simulink model "raspiAutopilotControlSystem"  (R2017b)
settings: Solver=ode5  StartTime=0.0  StopTime=inf  RelTol=1e-3  EnableMultiTasking=on
undefined symbols (not defined in the file): ap, env, sensors
libraries: etargetslib x2, simulink_extras x2, embdlinuxlib x2, mbdriLib x1
settings Model: ParamWorkspaceSource=ReferencedWorkspace  Creator=mlizarra  LastModifiedBy=mboyle
settings SolverCC: PositivePriorityOrder=on  AutoInsertRateTranBlk=on
settings DataIOCC: SaveOutput=off  DSMLogging=off  SaveTime=off  ReturnWorkspaceOutputs=on
settings OptimizationCC: DefaultParameterBehavior=Inlined  UseDivisionForNetSlopeComputation=UseDivisionForReciprocalsOfIntegersOnly  DefaultUnderspecifiedDataType=single  InlineInvariantSignals=on  PassReuseOutputArgsAs=Individual arguments  StateBitsets=on  DataBitsets=on  ZeroExternalMemoryAtStartup=off  ZeroInternalMemoryAtStartup=off  EfficientFloat2IntCast=on  LifeSpan=1  MaxStackSize=64
settings DebuggingCC: SignalInfNanChecking=warning  AlgebraicLoopMsg=error  ParameterPrecisionLossMsg=none  UniqueDataStoreMsg=error  AssertControl=DisableAll  SFUnexpectedBacktrackingDiag=warning  SFNoUnconditionalDefaultTransitionDiag=warning  SFExecutionAtInitializationDiag=none
settings HardwareCC: ProdBitPerPointer=32  ProdBitPerSizeT=32  ProdBitPerPtrDiffT=32  ProdLargestAtomicInteger=Long  ProdLargestAtomicFloat=Double  ProdWordSize=32  ProdHWDeviceType=ARM Compatible->ARM Cortex
settings SFSimCC: SimGenImportedTypeDefs=on  MATLABDynamicMemAlloc=off
settings RTWCC: SystemTargetFile=ert.tlc  HardwareBoard=Raspberry Pi  TemplateMakefile=ert_default_tmf  PostCodeGenCommand=add_header_files(h);  GenerateReport=on  CustomInclude=../src  Toolchain=GNU GCC Raspberry Pi  IncludeHyperlinkInReport=on  LaunchReport=on  PortableWordSizes=on  GenerateTraceInfo=on  GenerateTraceReport=on  GenerateTraceReportSl=on  GenerateTraceReportSf=on  GenerateTraceReportEml=on
settings CodeAppCC: ForceParamTrailComments=on  IgnoreCustomStorageClasses=off  IgnoreTestpoints=on  OperatorAnnotations=on  SimulinkDataObjDesc=on  SFDataObjDesc=on  MATLABFcnDesc=on  InsertBlockDesc=on  MATLABSourceComments=on
settings ERTTargetCC: TargetLangStandard=C99 (ISO)  CodeReplacementLibrary=GNU C99 extensions  SupportNonFinite=off  SupportVariableSizeSignals=on  InlinedParameterPlacement=NonHierarchical
settings ConfigComp: CovSaveCumulativeToWorkspaceVar=on

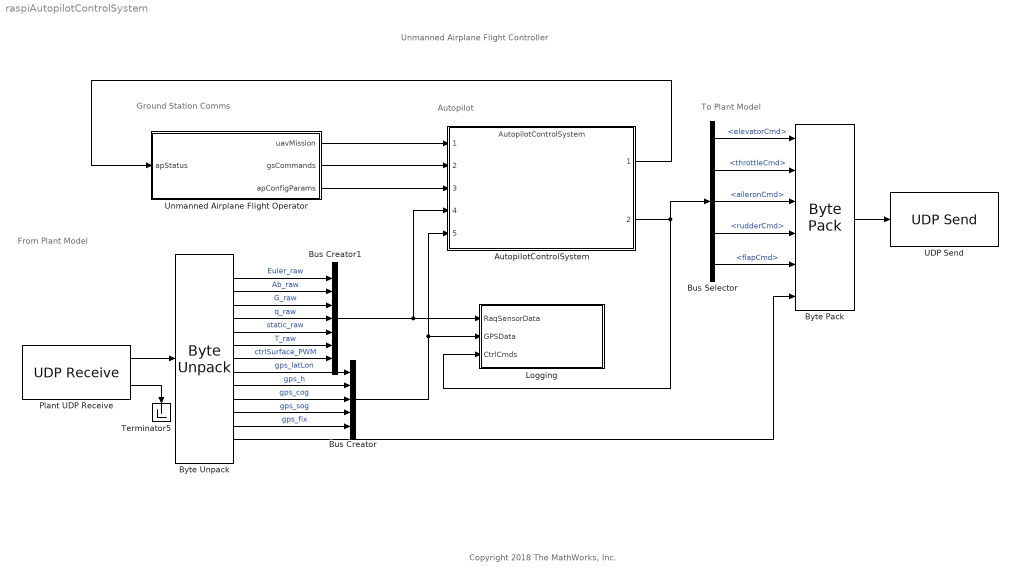
== system raspiAutopilotControlSystem ==
  note: To Plant Model
  note: From Plant Model
  note: Unmanned Airplane Flight Controller
  note: Ground Station Comms
  note: Autopilot
  note: Copyright 2018 The MathWorks, Inc.
  AutopilotControlSystem : ModelReference  ModelNameDialog=AutopilotControlSystem  SimulationMode=Normal  ModelReferenceVersion=1.356
  Bus Creator : BusCreator  Inputs=5  OutDataTypeStr=Bus: gpsReading
  Bus Creator1 : BusCreator  Inputs=7  OutDataTypeStr=Bus: rawSensorDataBus
  Bus Selector : BusSelector  OutputSignals=elevatorCmd,throttleCmd,aileronCmd,rudderCmd,flapCmd
  Byte Pack : etargetslib/Byte Pack  datatypes={'single', 'single','single', 'single','single','double'}  byteAlign=1
  Byte Unpack : etargetslib/Byte Unpack  dimensions={[3],[3],[3],1,1,1,[5],[2],1,1,1,1,1}  datatypes={'int16','int16','int16','uint16','uint16','int16','int16','single','single','single','single','uint8','double'}  byteAlign=1
  Logging : Subsystem
  Plant UDP Receive : embdlinuxlib/UDP Receive  localURL='0.0.0.0'  localPort=25001  remoteURL='0.0.0.0'  remotePort=-1  recvBufferSize=8192  signalDatatype=uint8  dims=63  isVarSize=off  showBlockingTime=off  blockingTime=0  sampletime=0.01  blockPlatform=Raspberry Pi
      settings: SourceProductName=Simulink Support Package for Raspberry Pi Hardware  SourceProductBaseCode=RASPPI
  Terminator5 : Terminator
  UDP Send : embdlinuxlib/UDP Send  remoteURL='10.10.10.6'  remotePort=25000  localURL='255.255.255.255'  localPortSource=Automatically determine  localPort=-1  sampletime=-1  blockPlatform=Raspberry Pi  separateLengthPort=0
      settings: SourceProductName=Simulink Support Package for Raspberry Pi Hardware  SourceProductBaseCode=RASPPI
  "Unmanned Airplane Flight Operator " : Subsystem
  wires:
  "Unmanned Airplane Flight Operator "/2(gsCommands) -> AutopilotControlSystem/2
  "Unmanned Airplane Flight Operator "/3(apConfigParams) -> AutopilotControlSystem/3
  AutopilotControlSystem/1 -> "Unmanned Airplane Flight Operator "/1(apStatus)
  "Unmanned Airplane Flight Operator "/1(uavMission) -> AutopilotControlSystem/1
  Plant UDP Receive/1 -> Byte Unpack/1
  Plant UDP Receive/2 -> Terminator5/1
  Byte Pack/1 -> UDP Send/1
  Bus Selector/1 -> Byte Pack/1  "<elevatorCmd>"
  Bus Selector/2 -> Byte Pack/2  "<throttleCmd>"
  Bus Selector/3 -> Byte Pack/3  "<aileronCmd>"
  Bus Selector/4 -> Byte Pack/4  "<rudderCmd>"
  Bus Selector/5 -> Byte Pack/5  "<flapCmd>"
  Byte Unpack/1 -> Bus Creator1/1  "Euler_raw"
  Byte Unpack/4 -> Bus Creator1/4  "q_raw"
  Byte Unpack/7 -> Bus Creator1/7  "ctrlSurface_PWM"
  Byte Unpack/6 -> Bus Creator1/6  "T_raw"
  Byte Unpack/3 -> Bus Creator1/3  "G_raw"
  Byte Unpack/5 -> Bus Creator1/5  "static_raw"
  Byte Unpack/2 -> Bus Creator1/2  "Ab_raw"
  Byte Unpack/12 -> Bus Creator/5  "gps_fix"
  Byte Unpack/11 -> Bus Creator/4  "gps_sog"
  Byte Unpack/10 -> Bus Creator/3  "gps_cog"
  Byte Unpack/9 -> Bus Creator/2  "gps_h"
  Byte Unpack/8 -> Bus Creator/1  "gps_latLon"
  Bus Creator1/1 -> AutopilotControlSystem/4, Logging/1(RaqSensorData)
  Bus Creator/1 -> AutopilotControlSystem/5, Logging/2(GPSData)
  AutopilotControlSystem/2 -> Logging/3(CtrlCmds), Bus Selector/1
  Byte Unpack/13 -> Byte Pack/6

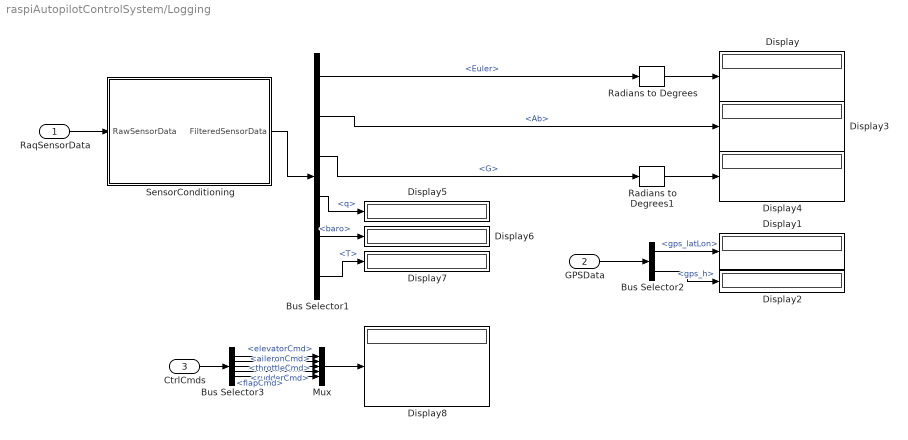
== system raspiAutopilotControlSystem/Logging ==
  RaqSensorData : Inport
  GPSData : Inport  Port=2
  CtrlCmds : Inport  Port=3
  Bus Selector1 : BusSelector  OutputSignals=Euler,Ab,G,q,baro,T
  Bus Selector2 : BusSelector  OutputSignals=gps_latLon,gps_h
  Bus Selector3 : BusSelector  OutputSignals=elevatorCmd,throttleCmd,aileronCmd,rudderCmd,flapCmd
  Display{,1..8} (9 alike) : Display
  Mux : Mux  Inputs=5
  Radians to Degrees : simulink_extras/Transformations/Radians to Degrees
  Radians to Degrees1 : simulink_extras/Transformations/Radians to Degrees
  SensorConditioning : Subsystem  TreatAsAtomicUnit=on
  wires:
  Bus Selector2/1 -> Display1/1  "<gps_latLon>"
  Bus Selector1/1 -> Radians to Degrees/1  "<Euler>"
  GPSData/1 -> Bus Selector2/1
  Bus Selector2/2 -> Display2/1  "<gps_h>"
  RaqSensorData/1 -> SensorConditioning/1(RawSensorData)
  SensorConditioning/1(FilteredSensorData) -> Bus Selector1/1
  Bus Selector1/2 -> Display3/1  "<Ab>"
  Bus Selector1/3 -> Radians to Degrees1/1  "<G>"
  Bus Selector1/4 -> Display5/1  "<q>"
  Bus Selector1/5 -> Display6/1  "<baro>"
  Bus Selector1/6 -> Display7/1  "<T>"
  Radians to Degrees/1 -> Display/1
  Radians to Degrees1/1 -> Display4/1
  CtrlCmds/1 -> Bus Selector3/1
  Bus Selector3/1 -> Mux/1  "<elevatorCmd>"
  Bus Selector3/2 -> Mux/2  "<throttleCmd>"
  Bus Selector3/3 -> Mux/3  "<aileronCmd>"
  Bus Selector3/4 -> Mux/4  "<rudderCmd>"
  Bus Selector3/5 -> Mux/5  "<flapCmd>"
  Mux/1 -> Display8/1

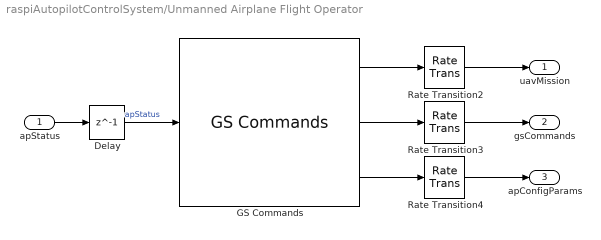
== system raspiAutopilotControlSystem/Unmanned Airplane Flight Operator  ==
  apStatus : Inport  OutDataTypeStr=Bus: apStatusBus
  Delay : Delay  DelayLength=1
  "GS Commands " : mbdriLib/Utilities/GS Commands 
  Rate Transition2 : RateTransition  OutPortSampleTime=ap.apSampleTime
  Rate Transition3 : RateTransition  OutPortSampleTime=ap.apSampleTime
  Rate Transition4 : RateTransition  OutPortSampleTime=ap.apSampleTime
  uavMission : Outport  OutDataTypeStr=Bus: waypoint
  gsCommands : Outport  Port=2  OutDataTypeStr=Bus: gsCommandsBus
  apConfigParams : Outport  Port=3  OutDataTypeStr=Bus: apConfigParamsBus
  wires:
  Rate Transition2/1 -> uavMission/1
  "GS Commands "/3 -> Rate Transition4/1
  apStatus/1 -> Delay/1
  "GS Commands "/2 -> Rate Transition3/1
  Delay/1 -> "GS Commands "/1  "apStatus"
  "GS Commands "/1 -> Rate Transition2/1
  Rate Transition4/1 -> apConfigParams/1
  Rate Transition3/1 -> gsCommands/1

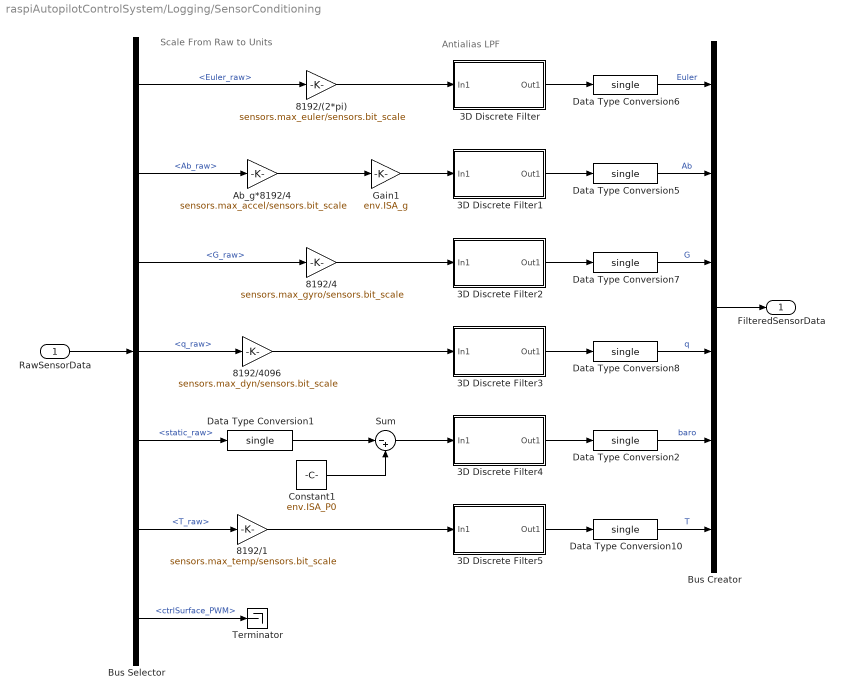
== system raspiAutopilotControlSystem/Logging/SensorConditioning ==
  note: Antialias LPF
  note: Scale From Raw to Units
  RawSensorData : Inport
  3D Discrete Filter : Subsystem  RTWFcnName=TustinFilter3D  mask{bw=sensors.antialiasBW, TSample=ap.apSampleTime}
      mask prompts: bw "Bandwith (Hz)"; TSample "Sample Time"
      mask init:
      | tau = 1/(2*pi*bw);
      | zval = [];
      | pval = -1/tau;
      | kval = 1/tau;
      | 
      | set_param(gcb,'AttributesFormatString', ['Fc = ' num2str(bw)]);
      settings: AttributesFormatString=Fc = 40  RTWFcnNameOpts=User specified  RTWFileNameOpts=Use function name
      mask Display:
      | droots(zval,pval,kval)
      | port_label('input',1,'3D')
  3D Discrete Filter1 : Subsystem  RTWFcnName=TustinFilter3D  mask{bw=sensors.antialiasBW, TSample=ap.apSampleTime}
      mask prompts: bw "Bandwith (Hz)"; TSample "Sample Time"
      mask init:
      | tau = 1/(2*pi*bw);
      | zval = [];
      | pval = -1/tau;
      | kval = 1/tau;
      | 
      | set_param(gcb,'AttributesFormatString', ['Fc = ' num2str(bw)]);
      settings: AttributesFormatString=Fc = 40  RTWFcnNameOpts=User specified  RTWFileNameOpts=Use function name
      mask Display:
      | droots(zval,pval,kval)
      | port_label('input',1,'3D')
  3D Discrete Filter2 : Subsystem  RTWFcnName=TustinFilter3D  mask{bw=sensors.antialiasBW, TSample=ap.apSampleTime}
      mask prompts: bw "Bandwith (Hz)"; TSample "Sample Time"
      mask init:
      | tau = 1/(2*pi*bw);
      | zval = [];
      | pval = -1/tau;
      | kval = 1/tau;
      | 
      | set_param(gcb,'AttributesFormatString', ['Fc = ' num2str(bw)]);
      settings: AttributesFormatString=Fc = 40  RTWFcnNameOpts=User specified  RTWFileNameOpts=Use function name
      mask Display:
      | droots(zval,pval,kval)
      | port_label('input',1,'3D')
  3D Discrete Filter3 : Subsystem  RTWFcnName=TustinFilter3D  mask{bw=sensors.antialiasBW, TSample=ap.apSampleTime}
      mask prompts: bw "Bandwith (Hz)"; TSample "Sample Time"
      mask init:
      | tau = 1/(2*pi*bw);
      | zval = [];
      | pval = -1/tau;
      | kval = 1/tau;
      | 
      | set_param(gcb,'AttributesFormatString', ['Fc = ' num2str(bw)]);
      settings: AttributesFormatString=Fc = 40  RTWFcnNameOpts=User specified  RTWFileNameOpts=Use function name
      mask Display:
      | droots(zval,pval,kval)
      | port_label('input',1,'1D')
  3D Discrete Filter4 : Subsystem  RTWFcnName=TustinFilter3D  mask{bw=sensors.antialiasBW, TSample=ap.apSampleTime}
      mask prompts: bw "Bandwith (Hz)"; TSample "Sample Time"
      mask init:
      | tau = 1/(2*pi*bw);
      | zval = [];
      | pval = -1/tau;
      | kval = 1/tau;
      | 
      | set_param(gcb,'AttributesFormatString', ['Fc = ' num2str(bw)]);
      settings: AttributesFormatString=Fc = 40  RTWFcnNameOpts=User specified  RTWFileNameOpts=Use function name
      mask Display:
      | droots(zval,pval,kval)
      | port_label('input',1,'1D')
  3D Discrete Filter5 : Subsystem  RTWFcnName=TustinFilter3D  mask{bw=sensors.antialiasBW, TSample=ap.apSampleTime}
      mask prompts: bw "Bandwith (Hz)"; TSample "Sample Time"
      mask init:
      | tau = 1/(2*pi*bw);
      | zval = [];
      | pval = -1/tau;
      | kval = 1/tau;
      | 
      | set_param(gcb,'AttributesFormatString', ['Fc = ' num2str(bw)]);
      settings: AttributesFormatString=Fc = 40  RTWFcnNameOpts=User specified  RTWFileNameOpts=Use function name
      mask Display:
      | droots(zval,pval,kval)
      | port_label('input',1,'1D')
  8192/(2*pi) : Gain  Gain=sensors.max_euler/sensors.bit_scale  OutDataTypeStr=single
      settings: AttributesFormatString=%<Gain>
  8192/1 : Gain  Gain=sensors.max_temp/sensors.bit_scale  OutDataTypeStr=single
      settings: AttributesFormatString=%<Gain>
  8192/4 : Gain  Gain=sensors.max_gyro/sensors.bit_scale  OutDataTypeStr=single
      settings: AttributesFormatString=%<Gain>
  8192/4096 : Gain  Gain=sensors.max_dyn/sensors.bit_scale  OutDataTypeStr=single
      settings: AttributesFormatString=%<Gain>
  Ab_g*8192/4 : Gain  Gain=sensors.max_accel/sensors.bit_scale  OutDataTypeStr=single
      settings: AttributesFormatString=%<Gain>
  Bus Creator : BusCreator  Inputs=6
  Bus Selector : BusSelector  OutputSignals=Euler_raw,Ab_raw,G_raw,q_raw,static_raw,T_raw,ctrlSurface_PWM
  Constant1 : Constant  Value=env.ISA_P0
      settings: AttributesFormatString=%<Value>
  Data Type Conversion{1..2,5..8,10} (7 alike) : DataTypeConversion  OutDataTypeStr=single
  Gain1 : Gain  Gain=env.ISA_g  OutDataTypeStr=single
      settings: AttributesFormatString=%<Gain>
  Sum : Sum  Inputs=|-+
  Terminator : Terminator
  FilteredSensorData : Outport
  wires:
  3D Discrete Filter5/1(Out1) -> Data Type Conversion10/1
  Data Type Conversion2/1 -> Bus Creator/5  "baro"
  3D Discrete Filter4/1(Out1) -> Data Type Conversion2/1
  3D Discrete Filter3/1(Out1) -> Data Type Conversion8/1
  3D Discrete Filter2/1(Out1) -> Data Type Conversion7/1
  3D Discrete Filter1/1(Out1) -> Data Type Conversion5/1
  3D Discrete Filter/1(Out1) -> Data Type Conversion6/1
  Data Type Conversion1/1 -> Sum/1
  Bus Creator/1 -> FilteredSensorData/1
  Gain1/1 -> 3D Discrete Filter1/1(In1)
  Bus Selector/2 -> Ab_g*8192/4/1  "<Ab_raw>"
  RawSensorData/1 -> Bus Selector/1
  Data Type Conversion6/1 -> Bus Creator/1  "Euler"
  Data Type Conversion5/1 -> Bus Creator/2  "Ab"
  Data Type Conversion7/1 -> Bus Creator/3  "G"
  Data Type Conversion8/1 -> Bus Creator/4  "q"
  Sum/1 -> 3D Discrete Filter4/1(In1)
  Data Type Conversion10/1 -> Bus Creator/6  "T"
  Constant1/1 -> Sum/2
  8192/1/1 -> 3D Discrete Filter5/1(In1)
  8192/4096/1 -> 3D Discrete Filter3/1(In1)
  Bus Selector/6 -> 8192/1/1  "<T_raw>"
  Bus Selector/5 -> Data Type Conversion1/1  "<static_raw>"
  Bus Selector/4 -> 8192/4096/1  "<q_raw>"
  Bus Selector/3 -> 8192/4/1  "<G_raw>"
  8192/4/1 -> 3D Discrete Filter2/1(In1)
  8192/(2*pi)/1 -> 3D Discrete Filter/1(In1)
  Ab_g*8192/4/1 -> Gain1/1
  Bus Selector/1 -> 8192/(2*pi)/1  "<Euler_raw>"
  Bus Selector/7 -> Terminator/1  "<ctrlSurface_PWM>"

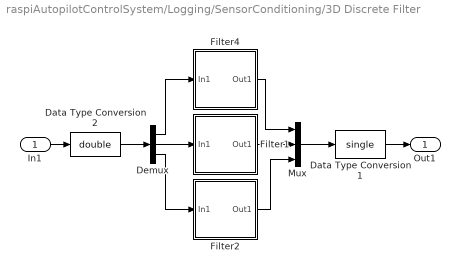
== system raspiAutopilotControlSystem/Logging/SensorConditioning/3D Discrete Filter ==
  In1 : Inport
  Data Type Conversion1 : DataTypeConversion  OutDataTypeStr=single
  Data Type Conversion2 : DataTypeConversion  OutDataTypeStr=double
  Demux : Demux  Outputs=3
  Filter1 : Subsystem  mask{Zeros=zval, Poles=pval, Gain=kval, AbsTol=auto, SampleTime=TSample, method=tustin, Wc=1}
      mask prompts: Zeros "Zeros (enter in s-main:)"; Poles "Poles (enter in s-domain:)"; Gain "Gain (enter in s-domain:)"; AbsTol "Absolute tolerance:"; SampleTime "Sample time:"; Wc "Critical Frequency (Hz):"
      mask init:
      | H = zpk(Zeros, Poles, Gain);
      | Hd = c2d(H, SampleTime, 'tustin');
      | [z, p, g] = zpkdata(Hd);
      | z_d = z{:};
      | p_d = p{:};
      | g_d = g;
      mask TypeOptions method: zoh | foh | tustin | prewarp | matched
      mask Display: droots(Zeros,Poles,Gain)
  Filter2 : Subsystem  mask{Zeros=zval, Poles=pval, Gain=kval, AbsTol=auto, SampleTime=TSample, method=tustin, Wc=1}
      mask prompts: Zeros "Zeros (enter in s-main:)"; Poles "Poles (enter in s-domain:)"; Gain "Gain (enter in s-domain:)"; AbsTol "Absolute tolerance:"; SampleTime "Sample time:"; Wc "Critical Frequency (Hz):"
      mask init:
      | H = zpk(Zeros, Poles, Gain);
      | Hd = c2d(H, SampleTime, 'tustin');
      | [z, p, g] = zpkdata(Hd);
      | z_d = z{:};
      | p_d = p{:};
      | g_d = g;
      mask TypeOptions method: zoh | foh | tustin | prewarp | matched
      mask Display: droots(Zeros,Poles,Gain)
  Filter4 : Subsystem  mask{Zeros=zval, Poles=pval, Gain=kval, AbsTol=auto, SampleTime=TSample, method=tustin, Wc=1}
      mask prompts: Zeros "Zeros (enter in s-main:)"; Poles "Poles (enter in s-domain:)"; Gain "Gain (enter in s-domain:)"; AbsTol "Absolute tolerance:"; SampleTime "Sample time:"; Wc "Critical Frequency (Hz):"
      mask init:
      | H = zpk(Zeros, Poles, Gain);
      | Hd = c2d(H, SampleTime, 'tustin');
      | [z, p, g] = zpkdata(Hd);
      | z_d = z{:};
      | p_d = p{:};
      | g_d = g;
      mask TypeOptions method: zoh | foh | tustin | prewarp | matched
      mask Display: droots(Zeros,Poles,Gain)
  Mux : Mux  Inputs=3
  Out1 : Outport
  wires:
  Data Type Conversion1/1 -> Out1/1
  Data Type Conversion2/1 -> Demux/1
  Demux/1 -> Filter4/1(In1)
  Demux/2 -> Filter1/1(In1)
  Demux/3 -> Filter2/1(In1)
  Filter4/1(Out1) -> Mux/1
  Filter1/1(Out1) -> Mux/2
  Filter2/1(Out1) -> Mux/3
  In1/1 -> Data Type Conversion2/1
  Mux/1 -> Data Type Conversion1/1

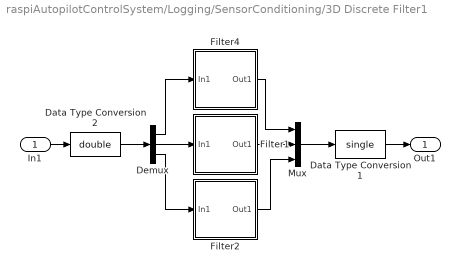
== system raspiAutopilotControlSystem/Logging/SensorConditioning/3D Discrete Filter1 ==
  In1 : Inport
  Data Type Conversion1 : DataTypeConversion  OutDataTypeStr=single
  Data Type Conversion2 : DataTypeConversion  OutDataTypeStr=double
  Demux : Demux  Outputs=3
  Filter1 : Subsystem  mask{Zeros=zval, Poles=pval, Gain=kval, AbsTol=auto, SampleTime=TSample, method=tustin, Wc=1}
      mask prompts: Zeros "Zeros (enter in s-main:)"; Poles "Poles (enter in s-domain:)"; Gain "Gain (enter in s-domain:)"; AbsTol "Absolute tolerance:"; SampleTime "Sample time:"; Wc "Critical Frequency (Hz):"
      mask init:
      | H = zpk(Zeros, Poles, Gain);
      | Hd = c2d(H, SampleTime, 'tustin');
      | [z, p, g] = zpkdata(Hd);
      | z_d = z{:};
      | p_d = p{:};
      | g_d = g;
      mask TypeOptions method: zoh | foh | tustin | prewarp | matched
      mask Display: droots(Zeros,Poles,Gain)
  Filter2 : Subsystem  mask{Zeros=zval, Poles=pval, Gain=kval, AbsTol=auto, SampleTime=TSample, method=tustin, Wc=1}
      mask prompts: Zeros "Zeros (enter in s-main:)"; Poles "Poles (enter in s-domain:)"; Gain "Gain (enter in s-domain:)"; AbsTol "Absolute tolerance:"; SampleTime "Sample time:"; Wc "Critical Frequency (Hz):"
      mask init:
      | H = zpk(Zeros, Poles, Gain);
      | Hd = c2d(H, SampleTime, 'tustin');
      | [z, p, g] = zpkdata(Hd);
      | z_d = z{:};
      | p_d = p{:};
      | g_d = g;
      mask TypeOptions method: zoh | foh | tustin | prewarp | matched
      mask Display: droots(Zeros,Poles,Gain)
  Filter4 : Subsystem  mask{Zeros=zval, Poles=pval, Gain=kval, AbsTol=auto, SampleTime=TSample, method=tustin, Wc=1}
      mask prompts: Zeros "Zeros (enter in s-main:)"; Poles "Poles (enter in s-domain:)"; Gain "Gain (enter in s-domain:)"; AbsTol "Absolute tolerance:"; SampleTime "Sample time:"; Wc "Critical Frequency (Hz):"
      mask init:
      | H = zpk(Zeros, Poles, Gain);
      | Hd = c2d(H, SampleTime, 'tustin');
      | [z, p, g] = zpkdata(Hd);
      | z_d = z{:};
      | p_d = p{:};
      | g_d = g;
      mask TypeOptions method: zoh | foh | tustin | prewarp | matched
      mask Display: droots(Zeros,Poles,Gain)
  Mux : Mux  Inputs=3
  Out1 : Outport
  wires:
  Mux/1 -> Data Type Conversion1/1
  In1/1 -> Data Type Conversion2/1
  Filter2/1(Out1) -> Mux/3
  Filter1/1(Out1) -> Mux/2
  Filter4/1(Out1) -> Mux/1
  Demux/3 -> Filter2/1(In1)
  Demux/2 -> Filter1/1(In1)
  Demux/1 -> Filter4/1(In1)
  Data Type Conversion2/1 -> Demux/1
  Data Type Conversion1/1 -> Out1/1

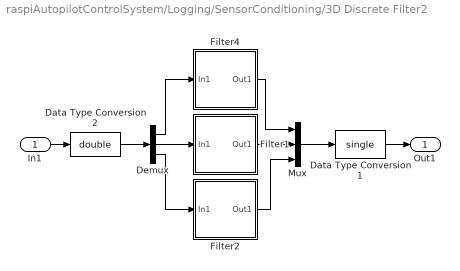
== system raspiAutopilotControlSystem/Logging/SensorConditioning/3D Discrete Filter2 ==
  In1 : Inport
  Data Type Conversion1 : DataTypeConversion  OutDataTypeStr=single
  Data Type Conversion2 : DataTypeConversion  OutDataTypeStr=double
  Demux : Demux  Outputs=3
  Filter1 : Subsystem  mask{Zeros=zval, Poles=pval, Gain=kval, AbsTol=auto, SampleTime=TSample, method=tustin, Wc=1}
      mask prompts: Zeros "Zeros (enter in s-main:)"; Poles "Poles (enter in s-domain:)"; Gain "Gain (enter in s-domain:)"; AbsTol "Absolute tolerance:"; SampleTime "Sample time:"; Wc "Critical Frequency (Hz):"
      mask init:
      | H = zpk(Zeros, Poles, Gain);
      | Hd = c2d(H, SampleTime, 'tustin');
      | [z, p, g] = zpkdata(Hd);
      | z_d = z{:};
      | p_d = p{:};
      | g_d = g;
      mask TypeOptions method: zoh | foh | tustin | prewarp | matched
      mask Display: droots(Zeros,Poles,Gain)
  Filter2 : Subsystem  mask{Zeros=zval, Poles=pval, Gain=kval, AbsTol=auto, SampleTime=TSample, method=tustin, Wc=1}
      mask prompts: Zeros "Zeros (enter in s-main:)"; Poles "Poles (enter in s-domain:)"; Gain "Gain (enter in s-domain:)"; AbsTol "Absolute tolerance:"; SampleTime "Sample time:"; Wc "Critical Frequency (Hz):"
      mask init:
      | H = zpk(Zeros, Poles, Gain);
      | Hd = c2d(H, SampleTime, 'tustin');
      | [z, p, g] = zpkdata(Hd);
      | z_d = z{:};
      | p_d = p{:};
      | g_d = g;
      mask TypeOptions method: zoh | foh | tustin | prewarp | matched
      mask Display: droots(Zeros,Poles,Gain)
  Filter4 : Subsystem  mask{Zeros=zval, Poles=pval, Gain=kval, AbsTol=auto, SampleTime=TSample, method=tustin, Wc=1}
      mask prompts: Zeros "Zeros (enter in s-main:)"; Poles "Poles (enter in s-domain:)"; Gain "Gain (enter in s-domain:)"; AbsTol "Absolute tolerance:"; SampleTime "Sample time:"; Wc "Critical Frequency (Hz):"
      mask init:
      | H = zpk(Zeros, Poles, Gain);
      | Hd = c2d(H, SampleTime, 'tustin');
      | [z, p, g] = zpkdata(Hd);
      | z_d = z{:};
      | p_d = p{:};
      | g_d = g;
      mask TypeOptions method: zoh | foh | tustin | prewarp | matched
      mask Display: droots(Zeros,Poles,Gain)
  Mux : Mux  Inputs=3
  Out1 : Outport
  wires:
  Data Type Conversion1/1 -> Out1/1
  Data Type Conversion2/1 -> Demux/1
  Demux/1 -> Filter4/1(In1)
  Demux/2 -> Filter1/1(In1)
  Demux/3 -> Filter2/1(In1)
  Filter4/1(Out1) -> Mux/1
  Filter1/1(Out1) -> Mux/2
  Filter2/1(Out1) -> Mux/3
  In1/1 -> Data Type Conversion2/1
  Mux/1 -> Data Type Conversion1/1

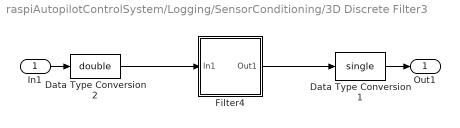
== system raspiAutopilotControlSystem/Logging/SensorConditioning/3D Discrete Filter3 ==
  In1 : Inport
  Data Type Conversion1 : DataTypeConversion  OutDataTypeStr=single
  Data Type Conversion2 : DataTypeConversion  OutDataTypeStr=double
  Filter4 : Subsystem  mask{Zeros=zval, Poles=pval, Gain=kval, AbsTol=auto, SampleTime=TSample, method=tustin, Wc=1}
      mask prompts: Zeros "Zeros (enter in s-main:)"; Poles "Poles (enter in s-domain:)"; Gain "Gain (enter in s-domain:)"; AbsTol "Absolute tolerance:"; SampleTime "Sample time:"; Wc "Critical Frequency (Hz):"
      mask init:
      | H = zpk(Zeros, Poles, Gain);
      | Hd = c2d(H, SampleTime, 'tustin');
      | [z, p, g] = zpkdata(Hd);
      | z_d = z{:};
      | p_d = p{:};
      | g_d = g;
      mask TypeOptions method: zoh | foh | tustin | prewarp | matched
      mask Display: droots(Zeros,Poles,Gain)
  Out1 : Outport
  wires:
  Filter4/1(Out1) -> Data Type Conversion1/1
  Data Type Conversion2/1 -> Filter4/1(In1)
  In1/1 -> Data Type Conversion2/1
  Data Type Conversion1/1 -> Out1/1

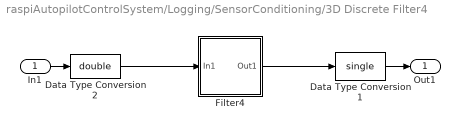
== system raspiAutopilotControlSystem/Logging/SensorConditioning/3D Discrete Filter4 ==
  In1 : Inport
  Data Type Conversion1 : DataTypeConversion  OutDataTypeStr=single
  Data Type Conversion2 : DataTypeConversion  OutDataTypeStr=double
  Filter4 : Subsystem  mask{Zeros=zval, Poles=pval, Gain=kval, AbsTol=auto, SampleTime=TSample, method=tustin, Wc=1}
      mask prompts: Zeros "Zeros (enter in s-main:)"; Poles "Poles (enter in s-domain:)"; Gain "Gain (enter in s-domain:)"; AbsTol "Absolute tolerance:"; SampleTime "Sample time:"; Wc "Critical Frequency (Hz):"
      mask init:
      | H = zpk(Zeros, Poles, Gain);
      | Hd = c2d(H, SampleTime, 'tustin');
      | [z, p, g] = zpkdata(Hd);
      | z_d = z{:};
      | p_d = p{:};
      | g_d = g;
      mask TypeOptions method: zoh | foh | tustin | prewarp | matched
      mask Display: droots(Zeros,Poles,Gain)
  Out1 : Outport
  wires:
  Data Type Conversion1/1 -> Out1/1
  In1/1 -> Data Type Conversion2/1
  Data Type Conversion2/1 -> Filter4/1(In1)
  Filter4/1(Out1) -> Data Type Conversion1/1

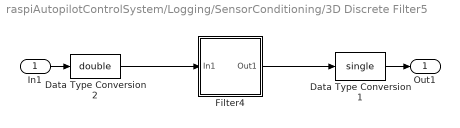
== system raspiAutopilotControlSystem/Logging/SensorConditioning/3D Discrete Filter5 ==
  In1 : Inport
  Data Type Conversion1 : DataTypeConversion  OutDataTypeStr=single
  Data Type Conversion2 : DataTypeConversion  OutDataTypeStr=double
  Filter4 : Subsystem  mask{Zeros=zval, Poles=pval, Gain=kval, AbsTol=auto, SampleTime=TSample, method=tustin, Wc=1}
      mask prompts: Zeros "Zeros (enter in s-main:)"; Poles "Poles (enter in s-domain:)"; Gain "Gain (enter in s-domain:)"; AbsTol "Absolute tolerance:"; SampleTime "Sample time:"; Wc "Critical Frequency (Hz):"
      mask init:
      | H = zpk(Zeros, Poles, Gain);
      | Hd = c2d(H, SampleTime, 'tustin');
      | [z, p, g] = zpkdata(Hd);
      | z_d = z{:};
      | p_d = p{:};
      | g_d = g;
      mask TypeOptions method: zoh | foh | tustin | prewarp | matched
      mask Display: droots(Zeros,Poles,Gain)
  Out1 : Outport
  wires:
  Filter4/1(Out1) -> Data Type Conversion1/1
  Data Type Conversion2/1 -> Filter4/1(In1)
  In1/1 -> Data Type Conversion2/1
  Data Type Conversion1/1 -> Out1/1

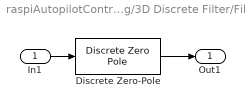
== system raspiAutopilotControlSystem/Logging/SensorConditioning/3D Discrete Filter/Filter1 ==
  In1 : Inport
  Discrete Zero-Pole : DiscreteZeroPole  Zeros=z_d  Poles=p_d  Gain=g_d  SampleTime=-1
  Out1 : Outport
  wires:
  In1/1 -> Discrete Zero-Pole/1
  Discrete Zero-Pole/1 -> Out1/1

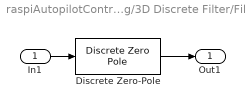
== system raspiAutopilotControlSystem/Logging/SensorConditioning/3D Discrete Filter/Filter2 ==
  In1 : Inport
  Discrete Zero-Pole : DiscreteZeroPole  Zeros=z_d  Poles=p_d  Gain=g_d  SampleTime=-1
  Out1 : Outport
  wires:
  Discrete Zero-Pole/1 -> Out1/1
  In1/1 -> Discrete Zero-Pole/1

== system raspiAutopilotControlSystem/Logging/SensorConditioning/3D Discrete Filter/Filter4 ==
  In1 : Inport
  Discrete Zero-Pole : DiscreteZeroPole  Zeros=z_d  Poles=p_d  Gain=g_d  SampleTime=-1
  Out1 : Outport
  wires:
  Discrete Zero-Pole/1 -> Out1/1
  In1/1 -> Discrete Zero-Pole/1

== system raspiAutopilotControlSystem/Logging/SensorConditioning/3D Discrete Filter1/Filter1 ==
  In1 : Inport
  Discrete Zero-Pole : DiscreteZeroPole  Zeros=z_d  Poles=p_d  Gain=g_d  SampleTime=-1
  Out1 : Outport
  wires:
  Discrete Zero-Pole/1 -> Out1/1
  In1/1 -> Discrete Zero-Pole/1

== system raspiAutopilotControlSystem/Logging/SensorConditioning/3D Discrete Filter1/Filter2 ==
  In1 : Inport
  Discrete Zero-Pole : DiscreteZeroPole  Zeros=z_d  Poles=p_d  Gain=g_d  SampleTime=-1
  Out1 : Outport
  wires:
  In1/1 -> Discrete Zero-Pole/1
  Discrete Zero-Pole/1 -> Out1/1

== system raspiAutopilotControlSystem/Logging/SensorConditioning/3D Discrete Filter1/Filter4 ==
  In1 : Inport
  Discrete Zero-Pole : DiscreteZeroPole  Zeros=z_d  Poles=p_d  Gain=g_d  SampleTime=-1
  Out1 : Outport
  wires:
  In1/1 -> Discrete Zero-Pole/1
  Discrete Zero-Pole/1 -> Out1/1

== system raspiAutopilotControlSystem/Logging/SensorConditioning/3D Discrete Filter2/Filter1 ==
  In1 : Inport
  Discrete Zero-Pole : DiscreteZeroPole  Zeros=z_d  Poles=p_d  Gain=g_d  SampleTime=-1
  Out1 : Outport
  wires:
  In1/1 -> Discrete Zero-Pole/1
  Discrete Zero-Pole/1 -> Out1/1

== system raspiAutopilotControlSystem/Logging/SensorConditioning/3D Discrete Filter2/Filter2 ==
  In1 : Inport
  Discrete Zero-Pole : DiscreteZeroPole  Zeros=z_d  Poles=p_d  Gain=g_d  SampleTime=-1
  Out1 : Outport
  wires:
  Discrete Zero-Pole/1 -> Out1/1
  In1/1 -> Discrete Zero-Pole/1

== system raspiAutopilotControlSystem/Logging/SensorConditioning/3D Discrete Filter2/Filter4 ==
  In1 : Inport
  Discrete Zero-Pole : DiscreteZeroPole  Zeros=z_d  Poles=p_d  Gain=g_d  SampleTime=-1
  Out1 : Outport
  wires:
  Discrete Zero-Pole/1 -> Out1/1
  In1/1 -> Discrete Zero-Pole/1

== system raspiAutopilotControlSystem/Logging/SensorConditioning/3D Discrete Filter3/Filter4 ==
  In1 : Inport
  Discrete Zero-Pole : DiscreteZeroPole  Zeros=z_d  Poles=p_d  Gain=g_d  SampleTime=-1
  Out1 : Outport
  wires:
  In1/1 -> Discrete Zero-Pole/1
  Discrete Zero-Pole/1 -> Out1/1

== system raspiAutopilotControlSystem/Logging/SensorConditioning/3D Discrete Filter4/Filter4 ==
  In1 : Inport
  Discrete Zero-Pole : DiscreteZeroPole  Zeros=z_d  Poles=p_d  Gain=g_d  SampleTime=-1
  Out1 : Outport
  wires:
  Discrete Zero-Pole/1 -> Out1/1
  In1/1 -> Discrete Zero-Pole/1

== system raspiAutopilotControlSystem/Logging/SensorConditioning/3D Discrete Filter5/Filter4 ==
  In1 : Inport
  Discrete Zero-Pole : DiscreteZeroPole  Zeros=z_d  Poles=p_d  Gain=g_d  SampleTime=-1
  Out1 : Outport
  wires:
  In1/1 -> Discrete Zero-Pole/1
  Discrete Zero-Pole/1 -> Out1/1
